simulink model "Microgrid_PV_WG_Bat_EV_j_22b"  (R2022b)
settings: Solver=VariableStepAuto  StartTime=0.0  StopTime=1  RelTol=1e-3
undefined symbols (not defined in the file or in its folder): Acid, Ion, Lead, Lithium
libraries: slpidlib x35, spsabctodq0Lib x23, spsSeriesRLCBranchLib x19, spsCurrentMeasurementLib x13, spsVoltageMeasurementLib x11, spsThreePhaseVIMeasurementLib x10, spsPLL3phLib x9, spsThreePhaseSeriesRLCBranchLib x9, spsPower3phInstantaneousLib x8, spsIGBTDiodeLib x8, spsUniversalBridgeLib x7, spsPWMGeneratorDCDCLib x6
(part 3 of 5)

== system Microgrid_PV_WG_Bat_EV_j_22b/Subsystem/电流内环控制，控制电网电流和电压同相 ==
  Id_ref : Inport
  Vd : Inport  Port=2
  Vq : Inport  Port=3
  f : Inport  Port=4
  Iq : Inport  Port=5
  Id : Inport  Port=6
  wt : Inport  Port=7
  Constant1 : Constant  Value=3e-3
  Constant2 : Constant  Value=0
  Constant3 : Constant  Value=0
  Constant4 : Constant  Value=3e-3
  Gain1 : Gain  Gain=2*pi
  Gain2 : Gain  Gain=2*pi
  Mux1 : Mux  Inputs=3
  PID Controller : slpidlib/PID Controller  Controller=PID  Form=Parallel  TimeDomain=Continuous-time  UseExternalTs=off  SampleTime=-1  IntegratorMethod=Forward Euler  FilterMethod=Forward Euler  ControllerParametersSource=internal  P=10  I=500  UseKiTs=off  D=0.5  N=100  UseFilter=on  TunerSelectOption=Transfer Function Based (PID Tuner App)  InitialConditionSource=internal  InitialConditionForIntegrator=0  InitialConditionForFilter=0  DifferentiatorICPrevScaledInput=0  ExternalReset=none  TrackingMode=off  Kt=1  LimitOutput=off  SatLimitsSource=internal  UpperSaturationLimit=inf  LowerSaturationLimit=-inf  LinearizeAsGain=on  AntiWindupMode=none  Kb=1  LimitIntegrator=off  UpperIntegratorSaturationLimit=inf  LowerIntegratorSaturationLimit=-inf  POutMin=[]  POutMax=[]  IOutMin=[]  IOutMax=[]  DOutMin=[]  DOutMax=[]  NOutMin=[]  NOutMax=[]  SumOutMin=[]  SumOutMax=[]  SaturationOutMin=[]  SaturationOutMax=[]  PParamMin=[]  PParamMax=[]  IParamMin=[]  IParamMax=[]  DParamMin=[]  DParamMax=[]  NParamMin=[]  NParamMax=[]  KbParamMin=[]  KbParamMax=[]  KtParamMin=[]  KtParamMax=[]  KbOutMin=[]  KbOutMax=[]  KtOutMin=[]  KtOutMax=[]  IntegratorOutMin=[]  IntegratorOutMax=[]  FilterOutMin=[]  FilterOutMax=[]  SumI1OutMin=[]  SumI1OutMax=[]  SumI2OutMin=[]  SumI2OutMax=[]  SumI3OutMin=[]  SumI3OutMax=[]  SumI4OutMin=[]  SumI4OutMax=[]  SumDOutMin=[]  SumDOutMax=[]  DifferentiatorOutMin=[]  DifferentiatorOutMax=[]  FilterDiffOutCoefMin=[]  FilterDiffOutCoefMax=[]  ReciprocalOutMin=[]  ReciprocalOutMax=[]  SumDenOutMin=[]  SumDenOutMax=[]  SumNumOutMin=[]  SumNumOutMax=[]  DivideOutMin=[]  DivideOutMax=[]  UdiffTsProdOutMin=[]  UdiffTsProdOutMax=[]  NTsProdOutMin=[]  NTsProdOutMax=[]  UintegralTsProdOutMin=[]  UintegralTsProdOutMax=[]  UngainTsProdOutMin=[]  UngainTsProdOutMax=[]  IntegratorContinuousStateAttributes=''  IntegratorStateMustResolveToSignalObject=off  IntegratorRTWStateStorageClass=Auto  FilterContinuousStateAttributes=''  FilterStateMustResolveToSignalObject=off  FilterRTWStateStorageClass=Auto  ParallelPVariant=InternalParameters  IdealPVariant=Disabled  IVariant=InternalParameters  DVariant=InternalParameters  IntegratorVariant=Continuous  SatVariant=Disabled  AWVariant=Passthrough  PCopyVariant=Disabled  TRVariant=Disabled  FdbkBlocksVariant=Forward  IdealPFdbkVariant=Disabled  SatFdbkVariant=Disabled  DerivativeFilterVariant=ContFilter  NVariant=InternalParameters  NCopyVariant=Disabled  FilterICVariant=InternalICsFilter  IntegratorICVariant=InternalICs  ExternalResetVariant=Disabled  TRSumVariant=Passthrough  SumFdbkVariant=Disabled  SumVariant=Sum_PID  TsampFilterVariant=InternalTs  TsampNgainVariant=Passthrough  TsampIntegralVariant=Disabled_SignalSpec  ExternalSaturationOutDataTypeStr=Inherit: Same as second input
  PID Controller1 : slpidlib/PID Controller  Controller=PID  Form=Parallel  TimeDomain=Continuous-time  UseExternalTs=off  SampleTime=-1  IntegratorMethod=Forward Euler  FilterMethod=Forward Euler  ControllerParametersSource=internal  P=10  I=500  UseKiTs=off  D=0.5  N=100  UseFilter=on  TunerSelectOption=Transfer Function Based (PID Tuner App)  InitialConditionSource=internal  InitialConditionForIntegrator=0  InitialConditionForFilter=0  DifferentiatorICPrevScaledInput=0  ExternalReset=none  TrackingMode=off  Kt=1  LimitOutput=off  SatLimitsSource=internal  UpperSaturationLimit=inf  LowerSaturationLimit=-inf  LinearizeAsGain=on  AntiWindupMode=none  Kb=1  LimitIntegrator=off  UpperIntegratorSaturationLimit=inf  LowerIntegratorSaturationLimit=-inf  POutMin=[]  POutMax=[]  IOutMin=[]  IOutMax=[]  DOutMin=[]  DOutMax=[]  NOutMin=[]  NOutMax=[]  SumOutMin=[]  SumOutMax=[]  SaturationOutMin=[]  SaturationOutMax=[]  PParamMin=[]  PParamMax=[]  IParamMin=[]  IParamMax=[]  DParamMin=[]  DParamMax=[]  NParamMin=[]  NParamMax=[]  KbParamMin=[]  KbParamMax=[]  KtParamMin=[]  KtParamMax=[]  KbOutMin=[]  KbOutMax=[]  KtOutMin=[]  KtOutMax=[]  IntegratorOutMin=[]  IntegratorOutMax=[]  FilterOutMin=[]  FilterOutMax=[]  SumI1OutMin=[]  SumI1OutMax=[]  SumI2OutMin=[]  SumI2OutMax=[]  SumI3OutMin=[]  SumI3OutMax=[]  SumI4OutMin=[]  SumI4OutMax=[]  SumDOutMin=[]  SumDOutMax=[]  DifferentiatorOutMin=[]  DifferentiatorOutMax=[]  FilterDiffOutCoefMin=[]  FilterDiffOutCoefMax=[]  ReciprocalOutMin=[]  ReciprocalOutMax=[]  SumDenOutMin=[]  SumDenOutMax=[]  SumNumOutMin=[]  SumNumOutMax=[]  DivideOutMin=[]  DivideOutMax=[]  UdiffTsProdOutMin=[]  UdiffTsProdOutMax=[]  NTsProdOutMin=[]  NTsProdOutMax=[]  UintegralTsProdOutMin=[]  UintegralTsProdOutMax=[]  UngainTsProdOutMin=[]  UngainTsProdOutMax=[]  IntegratorContinuousStateAttributes=''  IntegratorStateMustResolveToSignalObject=off  IntegratorRTWStateStorageClass=Auto  FilterContinuousStateAttributes=''  FilterStateMustResolveToSignalObject=off  FilterRTWStateStorageClass=Auto  ParallelPVariant=InternalParameters  IdealPVariant=Disabled  IVariant=InternalParameters  DVariant=InternalParameters  IntegratorVariant=Continuous  SatVariant=Disabled  AWVariant=Passthrough  PCopyVariant=Disabled  TRVariant=Disabled  FdbkBlocksVariant=Forward  IdealPFdbkVariant=Disabled  SatFdbkVariant=Disabled  DerivativeFilterVariant=ContFilter  NVariant=InternalParameters  NCopyVariant=Disabled  FilterICVariant=InternalICsFilter  IntegratorICVariant=InternalICs  ExternalResetVariant=Disabled  TRSumVariant=Passthrough  SumFdbkVariant=Disabled  SumVariant=Sum_PID  TsampFilterVariant=InternalTs  TsampNgainVariant=Passthrough  TsampIntegralVariant=Disabled_SignalSpec  ExternalSaturationOutDataTypeStr=Inherit: Same as second input
  PWM Generator (2-Level) : spsPWMGenerator2LevelLib/PWM Generator (2-Level)  ModulatorType=Three-phase bridge (6 pulses)  ModulatorMode=Unsynchronized  Fc=27*60  Pc=90  nF=27  MinMax="[ -1  1 ]"  SamplingTechnique=Natural  ModulatingSignals=off  m=0.8  Freq=60  Phase=0  Ts=0  ShowCarrierOutport=off
  Product{,1..3} (4 alike) : Product
  Subtract1 : Sum  Inputs=+-
  Subtract2 : Sum  Inputs=+-
  Sum : Sum  Inputs=+++
  Sum1 : Sum  Inputs=++-
  dq0 to abc : spsdq0toabcLib/dq0 to abc  Alignment=90 degrees behind phase A axis
  P : Outport
  wires:
  Gain2/1 -> Product2/1
  PWM Generator (2-Level)/1 -> P/1
  Constant4/1 -> Product2/2
  Mux1/1 -> dq0 to abc/1
  Sum/1 -> Mux1/1  "ud*"
  Id_ref/1 -> Subtract2/1
  Sum1/1 -> Mux1/2  "uq*"
  Product2/1 -> Product3/1
  dq0 to abc/1 -> PWM Generator (2-Level)/1
  Constant2/1 -> Subtract1/1  "iq*"
  Subtract2/1 -> PID Controller/1
  Constant3/1 -> Mux1/3
  PID Controller/1 -> Sum/2
  Vq/1 -> Sum1/1
  Product1/1 -> Sum/1
  Iq/1 -> Product1/2, Subtract1/2
  Constant1/1 -> Product/2
  f/1 -> Gain2/1, Gain1/1
  Gain1/1 -> Product/1
  wt/1 -> dq0 to abc/2
  Subtract1/1 -> PID Controller1/1
  Product3/1 -> Sum1/3
  PID Controller1/1 -> Sum1/2
  Product/1 -> Product1/1
  Id/1 -> Product3/2, Subtract2/2
  Vd/1 -> Sum/3

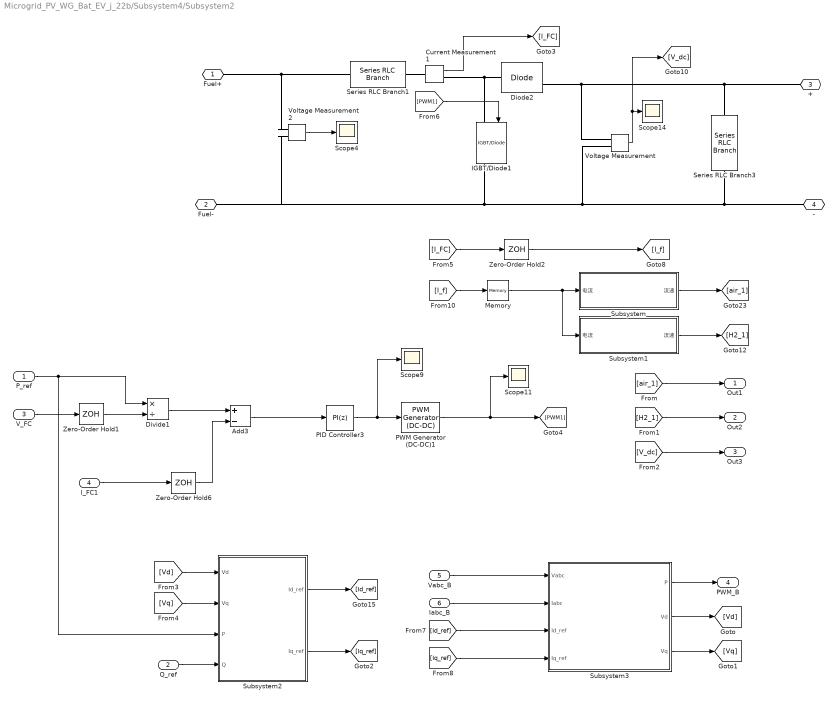
== system Microgrid_PV_WG_Bat_EV_j_22b/Subsystem4/Subsystem2 ==
  P_ref : Inport
  Q_ref : Inport  Port=2
  V_FC : Inport  Port=3
  I_FC1 : Inport  Port=4
  Vabc_B : Inport  Port=5
  Iabc_B : Inport  Port=6
  Add3 : Sum  Inputs=+-
  Current Measurement1 : spsCurrentMeasurementLib/Current Measurement  PhasorSimulation=off  OutputType=Complex  PSBequivalent=0
  Diode2 : spsDiodeLib/Diode  Ron=0.001  Lon=0  Vf=0.8  IC=0  UseSnubber=0  Rs=500  Cs=250e-9  Measurements=on
  Divide1 : Product  Inputs=*/
  IGBT/Diode1 : spsIGBTDiodeLib/IGBT//Diode  Ron=1e-3  Rs=1e5  Cs=inf  Measurements=on
  Memory : Memory  InitialCondition=1
  PID Controller3 : slpidlib/PID Controller  Controller=PI  Form=Parallel  TimeDomain=Discrete-time  UseExternalTs=off  SampleTime=-1  IntegratorMethod=Forward Euler  FilterMethod=Forward Euler  ControllerParametersSource=internal  P=1  I=1  UseKiTs=off  D=0  N=100  UseFilter=on  TunerSelectOption=Transfer Function Based (PID Tuner App)  InitialConditionSource=internal  InitialConditionForIntegrator=0  InitialConditionForFilter=0  DifferentiatorICPrevScaledInput=0  ExternalReset=none  TrackingMode=off  Kt=1  LimitOutput=off  SatLimitsSource=internal  UpperSaturationLimit=inf  LowerSaturationLimit=-inf  LinearizeAsGain=on  AntiWindupMode=none  Kb=1  LimitIntegrator=off  UpperIntegratorSaturationLimit=inf  LowerIntegratorSaturationLimit=-inf  POutMin=[]  POutMax=[]  IOutMin=[]  IOutMax=[]  DOutMin=[]  DOutMax=[]  NOutMin=[]  NOutMax=[]  SumOutMin=[]  SumOutMax=[]  SaturationOutMin=[]  SaturationOutMax=[]  PParamMin=[]  PParamMax=[]  IParamMin=[]  IParamMax=[]  DParamMin=[]  DParamMax=[]  NParamMin=[]  NParamMax=[]  KbParamMin=[]  KbParamMax=[]  KtParamMin=[]  KtParamMax=[]  KbOutMin=[]  KbOutMax=[]  KtOutMin=[]  KtOutMax=[]  IntegratorOutMin=[]  IntegratorOutMax=[]  FilterOutMin=[]  FilterOutMax=[]  SumI1OutMin=[]  SumI1OutMax=[]  SumI2OutMin=[]  SumI2OutMax=[]  SumI3OutMin=[]  SumI3OutMax=[]  SumI4OutMin=[]  SumI4OutMax=[]  SumDOutMin=[]  SumDOutMax=[]  DifferentiatorOutMin=[]  DifferentiatorOutMax=[]  FilterDiffOutCoefMin=[]  FilterDiffOutCoefMax=[]  ReciprocalOutMin=[]  ReciprocalOutMax=[]  SumDenOutMin=[]  SumDenOutMax=[]  SumNumOutMin=[]  SumNumOutMax=[]  DivideOutMin=[]  DivideOutMax=[]  UdiffTsProdOutMin=[]  UdiffTsProdOutMax=[]  NTsProdOutMin=[]  NTsProdOutMax=[]  UintegralTsProdOutMin=[]  UintegralTsProdOutMax=[]  UngainTsProdOutMin=[]  UngainTsProdOutMax=[]  IntegratorContinuousStateAttributes=''  IntegratorStateMustResolveToSignalObject=off  IntegratorRTWStateStorageClass=Auto  FilterContinuousStateAttributes=''  FilterStateMustResolveToSignalObject=off  FilterRTWStateStorageClass=Auto  ParallelPVariant=InternalParameters  IdealPVariant=Disabled  IVariant=InternalParameters  DVariant=Disabled  IntegratorVariant=Discrete  SatVariant=Disabled  AWVariant=Passthrough  PCopyVariant=Disabled  TRVariant=Disabled  FdbkBlocksVariant=Forward  IdealPFdbkVariant=Disabled  SatFdbkVariant=Disabled  DerivativeFilterVariant=Disabled  NVariant=Disabled  NCopyVariant=Disabled_SignalSpec  FilterICVariant=Disabled  IntegratorICVariant=InternalICs  ExternalResetVariant=Disabled  TRSumVariant=Passthrough  SumFdbkVariant=Disabled  SumVariant=Sum_PI  TsampFilterVariant=InternalTs  TsampNgainVariant=Passthrough  TsampIntegralVariant=Disabled_SignalSpec  ExternalSaturationOutDataTypeStr=Inherit: Same as second input
  PWM Generator (DC-DC)1 : spsPWMGeneratorDCDCLib/PWM Generator (DC-DC)  Fsw=1e4  Ts=0
  Scope{4,9,11,14} (4 alike) : Scope
  Series RLC Branch1 : spsSeriesRLCBranchLib/Series RLC Branch  LConnTagsString=__new0  RConnTagsString=__new0  BranchType=L  Resistance=1  Inductance=1e-2  SetiL0=off  InitialCurrent=0  Capacitance=1e-6  Setx0=off  InitialVoltage=0  Measurements=None
  Series RLC Branch3 : spsSeriesRLCBranchLib/Series RLC Branch  LConnTagsString=__new0  RConnTagsString=__new0  BranchType=C  Resistance=1  Inductance=1e-3  SetiL0=off  InitialCurrent=0  Capacitance=5e-2  Setx0=on  InitialVoltage=1000  Measurements=None
  Subsystem : Subsystem  mask{T=65, N=65, P=1.5, Uf_H2=99.56, x=99.95}
      mask prompts: T "温度"; N "数量"; P "氢气压强"; Uf_H2 "氢气利用率"; x "氢气百分比"
      mask DialogControl ParameterGroupVar Prompt: 参数
  Subsystem1 : Subsystem  mask{T=65, N=65, P=1, Uf_H2=59.3, x=21}
      mask prompts: T "温度"; N "数量"; P "氧气压强"; Uf_H2 "氧气利用率"; x "氧气百分比"
      mask DialogControl ParameterGroupVar Prompt: 参数
  Subsystem2 : Subsystem
  Subsystem3 : Subsystem
  Voltage Measurement : spsVoltageMeasurementLib/Voltage Measurement  PhasorSimulation=off  OutputType=Complex  PSBequivalent=0
  Voltage Measurement2 : spsVoltageMeasurementLib/Voltage Measurement  PhasorSimulation=off  OutputType=Complex  PSBequivalent=0
  Zero-Order Hold1 : ZeroOrderHold  SampleTime=1e-5
  Zero-Order Hold2 : ZeroOrderHold  SampleTime=1e-5
  Zero-Order Hold6 : ZeroOrderHold  SampleTime=1e-5
  Fuel+ : PMIOPort  Side=Left
  Fuel- : PMIOPort  Port=2  Side=Left
  + : PMIOPort  Port=3  Side=Right
  - : PMIOPort  Port=4  Side=Right
  Out1 : Outport
  Out2 : Outport  Port=2
  Out3 : Outport  Port=3
  PWM_B : Outport  Port=4
  wires:
  [PWM1] -> IGBT/Diode1/1
  Current Measurement1/1 -> [I_FC]
  Voltage Measurement/1 -> [V_dc], Scope14/1
  Voltage Measurement2/1 -> Scope4/1
  [I_FC] -> Zero-Order Hold2/1
  Zero-Order Hold2/1 -> [I_f]
  Subsystem/1(流速) -> [air_1]
  Subsystem1/1(流速) -> [H2_1]
  Memory/1 -> Subsystem1/1(电流), Subsystem/1(电流)
  [I_f] -> Memory/1
  [air_1] -> Out1/1
  [H2_1] -> Out2/1
  [V_dc] -> Out3/1
  Zero-Order Hold6/1 -> Add3/2
  Zero-Order Hold1/1 -> Divide1/2
  Divide1/1 -> Add3/1
  PWM Generator (DC-DC)1/1 -> Scope11/1, [PWM1]
  P_ref/1 -> Subsystem2/3(P), Divide1/1
  I_FC1/1 -> Zero-Order Hold6/1
  V_FC/1 -> Zero-Order Hold1/1
  Add3/1 -> PID Controller3/1
  PID Controller3/1 -> Scope9/1, PWM Generator (DC-DC)1/1
  Vabc_B/1 -> Subsystem3/1(Vabc)
  Iabc_B/1 -> Subsystem3/2(Iabc)
  Subsystem3/1(P) -> PWM_B/1
  Subsystem3/2(Vd) -> [Vd]
  Subsystem3/3(Vq) -> [Vq]
  [Vd] -> Subsystem2/1(Vd)
  [Vq] -> Subsystem2/2(Vq)
  Q_ref/1 -> Subsystem2/4(Q)
  Subsystem2/1(Id_ref) -> [Id_ref]
  Subsystem2/2(Iq_ref) -> [Iq_ref]
  [Id_ref] -> Subsystem3/3(Id_ref)
  [Iq_ref] -> Subsystem3/4(Iq_ref)
  connections:
  Current Measurement1/RConn1 -- IGBT/Diode1/LConn1 -- Diode2/LConn1
  Voltage Measurement2/LConn1 -- Fuel+/RConn1 -- Series RLC Branch1/LConn1
  Series RLC Branch3/LConn1 -- Voltage Measurement/LConn1 -- Diode2/RConn1 -- +/RConn1
  Current Measurement1/LConn1 -- Series RLC Branch1/RConn1
  IGBT/Diode1/RConn1 -- Voltage Measurement/LConn2 -- Series RLC Branch3/RConn1 -- -/RConn1 -- Voltage Measurement2/LConn2 -- Fuel-/RConn1

== system Microgrid_PV_WG_Bat_EV_j_22b/Subsystem4/Subsystem3 ==
  V_dc : Inport
  V_ref : Inport  Port=2
  Add1 : Sum  Inputs=+-
  Add4 : Sum  Inputs=+-
  Battery : spsBatteryLib/Battery  BatType=Lithium-Ion  ShowTempParam=off  ThermalPreset=no  ShowAgeParam=off  NomV=500  NomQ=100  SOC=50  Batt_Tr=30  PresetModel=on  MaxQ=100  MinV=375  FullV=581.9936  Dis_rate=43.4783  R=0.05  Normal_OP=90.4348  expZone="[540.1929      4.913043]"  current=[10 100]  Units=Time  Tci=20  NomT=20  T2=-30  MaxQ2=4.8  FullV2=7.1  Normal_OP2=5.655  expZone2="[6.58           1]"  Rca=0.6  ti=2000  Dp=0  Neq0=0  Tsim=1e6  Ta1=25  Qeol=5.4*0.9  Reol=0.013333*1.2  Char_age=[2.3478, 3]  Dis_age=[2.3478, 10]  N1=1500  N2=10500  N3=1000  N4=1400  Ta2=45  N5=950
  Current Measurement2 : spsCurrentMeasurementLib/Current Measurement  PhasorSimulation=off  OutputType=Complex  PSBequivalent=0
  Demux : Demux  Outputs=3
  IGBT/Diode2 : spsIGBTDiodeLib/IGBT//Diode  Ron=1e-3  Rs=1e5  Cs=inf  Measurements=on
  IGBT/Diode3 : spsIGBTDiodeLib/IGBT//Diode  Ron=1e-3  Rs=1e5  Cs=inf  Measurements=on
  NOT : Logic  Operator=NOT  IconShape=distinctive  AllPortsSameDT=off  OutDataTypeStr=boolean
  PID Controller2 : slpidlib/PID Controller  Controller=PI  Form=Parallel  TimeDomain=Continuous-time  UseExternalTs=off  SampleTime=-1  IntegratorMethod=Forward Euler  FilterMethod=Forward Euler  ControllerParametersSource=internal  P=10  I=1000  UseKiTs=off  D=0  N=100  UseFilter=on  TunerSelectOption=Transfer Function Based (PID Tuner App)  InitialConditionSource=internal  InitialConditionForIntegrator=0  InitialConditionForFilter=0  DifferentiatorICPrevScaledInput=0  ExternalReset=none  TrackingMode=off  Kt=1  LimitOutput=off  SatLimitsSource=internal  UpperSaturationLimit=inf  LowerSaturationLimit=-inf  LinearizeAsGain=on  AntiWindupMode=none  Kb=1  LimitIntegrator=off  UpperIntegratorSaturationLimit=inf  LowerIntegratorSaturationLimit=-inf  POutMin=[]  POutMax=[]  IOutMin=[]  IOutMax=[]  DOutMin=[]  DOutMax=[]  NOutMin=[]  NOutMax=[]  SumOutMin=[]  SumOutMax=[]  SaturationOutMin=[]  SaturationOutMax=[]  PParamMin=[]  PParamMax=[]  IParamMin=[]  IParamMax=[]  DParamMin=[]  DParamMax=[]  NParamMin=[]  NParamMax=[]  KbParamMin=[]  KbParamMax=[]  KtParamMin=[]  KtParamMax=[]  KbOutMin=[]  KbOutMax=[]  KtOutMin=[]  KtOutMax=[]  IntegratorOutMin=[]  IntegratorOutMax=[]  FilterOutMin=[]  FilterOutMax=[]  SumI1OutMin=[]  SumI1OutMax=[]  SumI2OutMin=[]  SumI2OutMax=[]  SumI3OutMin=[]  SumI3OutMax=[]  SumI4OutMin=[]  SumI4OutMax=[]  SumDOutMin=[]  SumDOutMax=[]  DifferentiatorOutMin=[]  DifferentiatorOutMax=[]  FilterDiffOutCoefMin=[]  FilterDiffOutCoefMax=[]  ReciprocalOutMin=[]  ReciprocalOutMax=[]  SumDenOutMin=[]  SumDenOutMax=[]  SumNumOutMin=[]  SumNumOutMax=[]  DivideOutMin=[]  DivideOutMax=[]  UdiffTsProdOutMin=[]  UdiffTsProdOutMax=[]  NTsProdOutMin=[]  NTsProdOutMax=[]  UintegralTsProdOutMin=[]  UintegralTsProdOutMax=[]  UngainTsProdOutMin=[]  UngainTsProdOutMax=[]  IntegratorContinuousStateAttributes=''  IntegratorStateMustResolveToSignalObject=off  IntegratorRTWStateStorageClass=Auto  FilterContinuousStateAttributes=''  FilterStateMustResolveToSignalObject=off  FilterRTWStateStorageClass=Auto  ParallelPVariant=InternalParameters  IdealPVariant=Disabled  IVariant=InternalParameters  DVariant=Disabled  IntegratorVariant=Continuous  SatVariant=Disabled  AWVariant=Passthrough  PCopyVariant=Disabled  TRVariant=Disabled  FdbkBlocksVariant=Forward  IdealPFdbkVariant=Disabled  SatFdbkVariant=Disabled  DerivativeFilterVariant=Disabled  NVariant=Disabled  NCopyVariant=Disabled_SignalSpec  FilterICVariant=Disabled  IntegratorICVariant=InternalICs  ExternalResetVariant=Disabled  TRSumVariant=Passthrough  SumFdbkVariant=Disabled  SumVariant=Sum_PI  TsampFilterVariant=InternalTs  TsampNgainVariant=Passthrough  TsampIntegralVariant=Disabled_SignalSpec  ExternalSaturationOutDataTypeStr=Inherit: Same as second input
  PID Controller4 : slpidlib/PID Controller  Controller=PI  Form=Parallel  TimeDomain=Continuous-time  UseExternalTs=off  SampleTime=-1  IntegratorMethod=Forward Euler  FilterMethod=Forward Euler  ControllerParametersSource=internal  P=1  I=1  UseKiTs=off  D=0  N=100  UseFilter=on  TunerSelectOption=Transfer Function Based (PID Tuner App)  InitialConditionSource=internal  InitialConditionForIntegrator=0  InitialConditionForFilter=0  DifferentiatorICPrevScaledInput=0  ExternalReset=none  TrackingMode=off  Kt=1  LimitOutput=off  SatLimitsSource=internal  UpperSaturationLimit=inf  LowerSaturationLimit=-inf  LinearizeAsGain=on  AntiWindupMode=none  Kb=1  LimitIntegrator=off  UpperIntegratorSaturationLimit=inf  LowerIntegratorSaturationLimit=-inf  POutMin=[]  POutMax=[]  IOutMin=[]  IOutMax=[]  DOutMin=[]  DOutMax=[]  NOutMin=[]  NOutMax=[]  SumOutMin=[]  SumOutMax=[]  SaturationOutMin=[]  SaturationOutMax=[]  PParamMin=[]  PParamMax=[]  IParamMin=[]  IParamMax=[]  DParamMin=[]  DParamMax=[]  NParamMin=[]  NParamMax=[]  KbParamMin=[]  KbParamMax=[]  KtParamMin=[]  KtParamMax=[]  KbOutMin=[]  KbOutMax=[]  KtOutMin=[]  KtOutMax=[]  IntegratorOutMin=[]  IntegratorOutMax=[]  FilterOutMin=[]  FilterOutMax=[]  SumI1OutMin=[]  SumI1OutMax=[]  SumI2OutMin=[]  SumI2OutMax=[]  SumI3OutMin=[]  SumI3OutMax=[]  SumI4OutMin=[]  SumI4OutMax=[]  SumDOutMin=[]  SumDOutMax=[]  DifferentiatorOutMin=[]  DifferentiatorOutMax=[]  FilterDiffOutCoefMin=[]  FilterDiffOutCoefMax=[]  ReciprocalOutMin=[]  ReciprocalOutMax=[]  SumDenOutMin=[]  SumDenOutMax=[]  SumNumOutMin=[]  SumNumOutMax=[]  DivideOutMin=[]  DivideOutMax=[]  UdiffTsProdOutMin=[]  UdiffTsProdOutMax=[]  NTsProdOutMin=[]  NTsProdOutMax=[]  UintegralTsProdOutMin=[]  UintegralTsProdOutMax=[]  UngainTsProdOutMin=[]  UngainTsProdOutMax=[]  IntegratorContinuousStateAttributes=''  IntegratorStateMustResolveToSignalObject=off  IntegratorRTWStateStorageClass=Auto  FilterContinuousStateAttributes=''  FilterStateMustResolveToSignalObject=off  FilterRTWStateStorageClass=Auto  ParallelPVariant=InternalParameters  IdealPVariant=Disabled  IVariant=InternalParameters  DVariant=Disabled  IntegratorVariant=Continuous  SatVariant=Disabled  AWVariant=Passthrough  PCopyVariant=Disabled  TRVariant=Disabled  FdbkBlocksVariant=Forward  IdealPFdbkVariant=Disabled  SatFdbkVariant=Disabled  DerivativeFilterVariant=Disabled  NVariant=Disabled  NCopyVariant=Disabled_SignalSpec  FilterICVariant=Disabled  IntegratorICVariant=InternalICs  ExternalResetVariant=Disabled  TRSumVariant=Passthrough  SumFdbkVariant=Disabled  SumVariant=Sum_PI  TsampFilterVariant=InternalTs  TsampNgainVariant=Passthrough  TsampIntegralVariant=Disabled_SignalSpec  ExternalSaturationOutDataTypeStr=Inherit: Same as second input
  PWM Generator (DC-DC)2 : spsPWMGeneratorDCDCLib/PWM Generator (DC-DC)  Fsw=1e4  Ts=0
  Scope : Scope  NumInputPorts=3
  Series RLC Branch4 : spsSeriesRLCBranchLib/Series RLC Branch  LConnTagsString=__new0  RConnTagsString=__new0  BranchType=L  Resistance=1  Inductance=1e-3  SetiL0=off  InitialCurrent=0  Capacitance=1e-6  Setx0=off  InitialVoltage=0  Measurements=None
  Series RLC Branch5 : spsSeriesRLCBranchLib/Series RLC Branch  LConnTagsString=__new0  RConnTagsString=__new0  BranchType=C  Resistance=1  Inductance=1e-3  SetiL0=off  InitialCurrent=0  Capacitance=1e-3  Setx0=off  InitialVoltage=0  Measurements=None
  Series RLC Branch6 : spsSeriesRLCBranchLib/Series RLC Branch  LConnTagsString=__new0  RConnTagsString=__new0  BranchType=R  Resistance=1  Inductance=1e-3  SetiL0=off  InitialCurrent=0  Capacitance=1e-6  Setx0=off  InitialVoltage=0  Measurements=None
  Zero-Order Hold4 : ZeroOrderHold  SampleTime=1e-5
  Zero-Order Hold5 : ZeroOrderHold  SampleTime=1e-5
  Bat+ : PMIOPort  Side=Left
  Bat- : PMIOPort  Port=2  Side=Left
  Out1 : Outport
  wires:
  Current Measurement2/1 -> [I_BA]
  [PWM2] -> IGBT/Diode2/1
  [PWM3] -> IGBT/Diode3/1
  PID Controller2/1 -> Add4/1
  Add1/1 -> PID Controller2/1
  Zero-Order Hold5/1 -> Add1/1
  PWM Generator (DC-DC)2/1 -> NOT/1, [PWM2]
  PID Controller4/1 -> PWM Generator (DC-DC)2/1
  Add4/1 -> PID Controller4/1
  NOT/1 -> [PWM3]
  V_ref/1 -> Add1/2
  [I_BA] -> Zero-Order Hold4/1
  Zero-Order Hold4/1 -> Add4/2
  V_dc/1 -> Zero-Order Hold5/1
  Battery/1 -> Demux/1
  Demux/1 -> Scope/1
  Demux/2 -> Scope/2
  Demux/3 -> Scope/3
  connections:
  Current Measurement2/RConn1 -- Battery/LConn1 -- Series RLC Branch6/LConn1
  IGBT/Diode3/RConn1 -- Series RLC Branch5/RConn1 -- Battery/LConn2 -- Series RLC Branch6/RConn1 -- Bat-/RConn1
  IGBT/Diode3/LConn1 -- IGBT/Diode2/RConn1 -- Series RLC Branch4/LConn1
  Series RLC Branch5/LConn1 -- Current Measurement2/LConn1 -- Series RLC Branch4/RConn1
  IGBT/Diode2/LConn1 -- Bat+/RConn1

== system Microgrid_PV_WG_Bat_EV_j_22b/储氢罐/氢气消耗速率转换 ==
  L/min : Inport
  Add : Sum
  Divide : Product  Inputs=*/
  Gain : Gain  Gain=1/60/1000
  P : Constant  Value=101325
  Product : Product
  Product1 : Product
  R : Constant  Value=8.314
  T/C : Constant  Value=25
  conversion : Constant  Value=273.15
  mol/s : Outport
  wires:
  P/1 -> Product/2
  conversion/1 -> Add/2
  T/C/1 -> Add/1
  R/1 -> Product1/1
  Add/1 -> Product1/2  "T/K"
  Product/1 -> Divide/1
  L/min/1 -> Gain/1
  Product1/1 -> Divide/2
  Gain/1 -> Product/1
  Divide/1 -> mol/s/1

== system Microgrid_PV_WG_Bat_EV_j_22b/充电桩/恒流恒压充电 ==
  V : Inport
  I : Inport  Port=2
  Add : Sum
  Constant : Constant
  Constant1 : Constant  Value=0
  Constant2 : Constant
  Memory : Memory
  Memory1 : Memory  InitialCondition=0.3
  Saturation : Saturate  UpperLimit=1  LowerLimit=0
  Sign : Signum
  Sum1 : Sum  Inputs=|++
  Sum2 : Sum  Inputs=|-+
  Switch : Switch  Threshold=500  SaturateOnIntegerOverflow=off  InputSameDT=off
  恒压 : Subsystem
  恒流 : Subsystem
  D : Outport
  wires:
  V/1 -> Switch/2, 恒压/1(V)
  恒压/1(I_out) -> Add/2
  I/1 -> 恒流/1(I)
  Add/1 -> Saturation/1
  Saturation/1 -> Memory1/1
  Constant/1 -> Switch/1
  Constant1/1 -> Switch/3
  Sum1/1 -> Memory/1
  Memory/1 -> Sign/1
  Sign/1 -> Sum2/1, 恒压/Enable, Sum1/2
  Switch/1 -> Sum1/1
  Constant2/1 -> Sum2/2
  Sum2/1 -> 恒流/Enable
  恒流/1(I_out) -> Add/1
  Memory1/1 -> D/1

== system Microgrid_PV_WG_Bat_EV_j_22b/光伏/电导增量法MPPT ==
  V : Inport
  I : Inport  Port=2
  Add : Sum
  Add1 : Sum
  Constant : Constant  Value=0
  Constant1 : Constant  Value=0
  Gain : Gain  Gain=-2e-6
  Gain1 : Gain  Gain=-2e-6
  Math Function : Math  Operator=square
  Memory : Memory
  Memory1 : Memory
  Memory2 : Memory  InitialCondition=0.5
  Product : Product  Inputs=3
  Product1 : Product
  Sign : Signum
  Sign1 : Signum
  Subtract : Sum  Inputs=+-
  Switch : Switch  Criteria=u2 ~= 0  SaturateOnIntegerOverflow=off  InputSameDT=off
  Switch1 : Switch  Criteria=u2 ~= 0  SaturateOnIntegerOverflow=off  InputSameDT=off
  Switch2 : Switch  Criteria=u2 ~= 0  SaturateOnIntegerOverflow=off  InputSameDT=off
  计算电流变化量 : Sum  Inputs=+-
  D : Outport
  wires:
  V/1 -> Product/3, Memory1/1, Subtract/1
  Memory/1 -> 计算电流变化量/2
  Memory1/1 -> Subtract/2
  Switch/1 -> Add/1
  Add/1 -> D/1, Memory2/1  "过程量转为状态量"
  Memory2/1 -> Add/2
  I/1 -> Product1/2, Memory/1, 计算电流变化量/1
  Subtract/1 -> Switch/2, Product/1, Math Function/1  "dV"
  Math Function/1 -> Product1/1
  计算电流变化量/1 -> Sign1/1, Product/2, Switch2/2  "dI"
  Product1/1 -> Add1/1
  Product/1 -> Add1/2
  Add1/1 -> Sign/1, Switch1/2  "I+dI/dV*V"
  Constant/1 -> Switch1/3
  Sign/1 -> Gain/1
  Gain/1 -> Switch1/1
  Switch1/1 -> Switch/1
  Constant1/1 -> Switch2/3
  Sign1/1 -> Gain1/1
  Gain1/1 -> Switch2/1
  Switch2/1 -> Switch/3

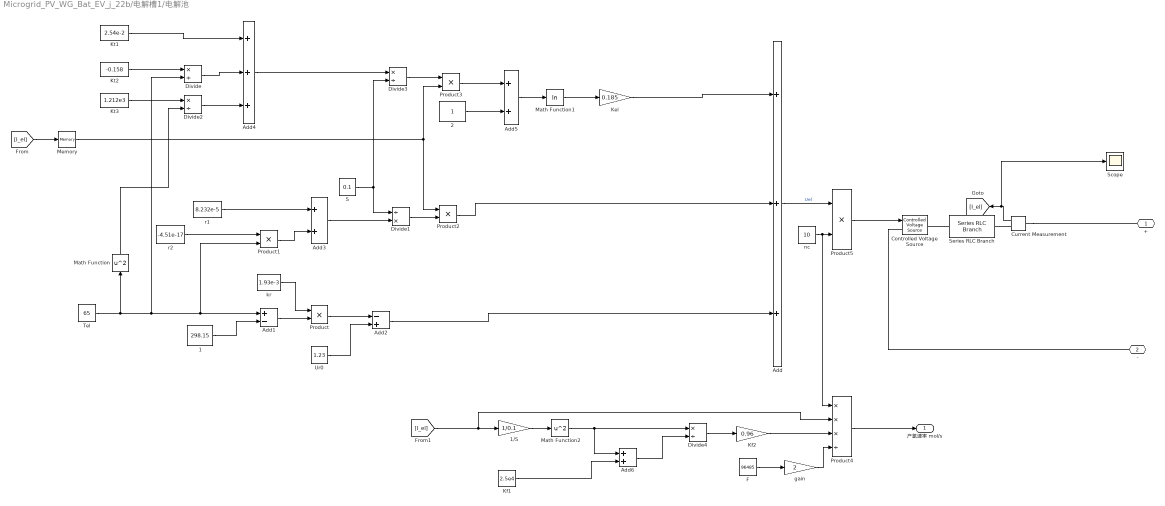
== system Microgrid_PV_WG_Bat_EV_j_22b/电解槽1/电解池 ==
  1 : Constant  Value=298.15
  1/S : Gain  Gain=1/0.1
  2 : Constant
  Add : Sum  Inputs=+++
  Add1 : Sum  Inputs=+-
  Add2 : Sum  Inputs=-+
  Add3 : Sum
  Add4 : Sum  Inputs=+++
  Add5 : Sum
  Add6 : Sum
  Controlled Voltage Source : spsControlledVoltageSourceLib/Controlled Voltage Source  Initialize=on  Source_Type=AC  Amplitude=0  Phase=0  Frequency=0  Measurements=None
  Current Measurement : spsCurrentMeasurementLib/Current Measurement  PhasorSimulation=off  OutputType=Complex  PSBequivalent=0
  Divide{,2..4} (4 alike) : Product  Inputs=*/
  Divide1 : Product  Inputs=/*
  F : Constant  Value=96485
  Kel : Gain  Gain=0.185
  Kf1 : Constant  Value=2.5e4
  Kf2 : Gain  Gain=0.96
  Kt1 : Constant  Value=2.54e-2
  Kt2 : Constant  Value=-0.158
  Kt3 : Constant  Value=1.212e3
  Math Function : Math  Operator=square
  Math Function1 : Math  Operator=log
  Math Function2 : Math  Operator=square
  Memory : Memory  InitialCondition=10
  Product{,1..3,5} (5 alike) : Product
  Product4 : Product  Inputs=***/
  S : Constant  Value=0.1
  Scope : Scope
  Series RLC Branch : spsSeriesRLCBranchLib/Series RLC Branch  LConnTagsString=__new0  RConnTagsString=__new0  BranchType=R  Resistance=1  Inductance=1e-3  SetiL0=off  InitialCurrent=0  Capacitance=1e-6  Setx0=off  InitialVoltage=0  Measurements=None
  Tel : Constant  Value=65
  Ur0 : Constant  Value=1.23
  gain : Gain  Gain=2
  kr : Constant  Value=1.93e-3
  nc : Constant  Value=10
  r1 : Constant  Value=8.232e-5
  r2 : Constant  Value=-4.51e-17
  + : PMIOPort  Side=Left
  - : PMIOPort  Port=2  Side=Left
  产氢速率 mol/s : Outport
  wires:
  Add3/1 -> Divide1/2
  Kt2/1 -> Divide/1
  Divide3/1 -> Product3/1
  Tel/1 -> Math Function/1, Divide/2, Product1/2, Add1/1
  [I_el] -> Memory/1
  Add5/1 -> Math Function1/1
  S/1 -> Divide3/2, Divide1/1
  Current Measurement/1 -> Scope/1, [I_el]
  r2/1 -> Product1/1
  Product1/1 -> Add3/2
  Product/1 -> Add2/1
  Math Function1/1 -> Kel/1
  1/1 -> Add1/2
  2/1 -> Add5/2
  r1/1 -> Add3/1
  Divide/1 -> Add4/2
  Add2/1 -> Add/3
  Kel/1 -> Add/1
  Add4/1 -> Divide3/1
  Product2/1 -> Add/2
  Kt3/1 -> Divide2/1
  Math Function/1 -> Divide2/2
  Kt1/1 -> Add4/1
  Divide2/1 -> Add4/3
  Ur0/1 -> Add2/2
  Divide1/1 -> Product2/2
  Product3/1 -> Add5/1
  Add1/1 -> Product/2
  kr/1 -> Product/1
  Add/1 -> Product5/1  "Uel"
  1/S/1 -> Math Function2/1
  Kf1/1 -> Add6/2
  Math Function2/1 -> Divide4/1, Add6/1
  Add6/1 -> Divide4/2
  [I_el] -> Product4/2, 1/S/1
  Divide4/1 -> Kf2/1
  Kf2/1 -> Product4/3
  nc/1 -> Product4/1, Product5/2
  Product5/1 -> Controlled Voltage Source/1
  F/1 -> gain/1
  gain/1 -> Product4/4
  Product4/1 -> 产氢速率 mol/s/1
  Memory/1 -> Product3/2, Product2/1
  connections:
  Controlled Voltage Source/LConn1 -- -/RConn1
  Series RLC Branch/LConn1 -- Controlled Voltage Source/RConn1
  Current Measurement/RConn1 -- Series RLC Branch/RConn1
  Current Measurement/LConn1 -- +/RConn1

== system Microgrid_PV_WG_Bat_EV_j_22b/逆变器整流/controller2 ==
  note: abc2dq
  Udc : Inport
  Udc_ref : Inport  Port=2
  Vabc : Inport  Port=3
  Iabc : Inport  Port=4
  Constant : Constant  Commented=on  Value=600
  Constant4 : Constant  Value=0
  Demux2 : Demux  Outputs=3
  Demux3 : Demux  Outputs=3
  Demux4 : Demux  Outputs=3
  Gain6 : Gain  Gain=2*pi*50*(7e-3)
  Gain7 : Gain  Gain=2*pi*50*(7e-3)
  Gain9 : Gain  Gain=0.0017
  Mux1 : Mux  Inputs=3
  PID 3 : slpidlib/PID Controller  Controller=PID  Form=Parallel  TimeDomain=Discrete-time  UseExternalTs=off  SampleTime=1e-5  IntegratorMethod=Forward Euler  FilterMethod=Forward Euler  ControllerParametersSource=internal  P=2  I=70  UseKiTs=off  D=0  N=100  UseFilter=on  TunerSelectOption=Transfer Function Based (PID Tuner App)  InitialConditionSource=internal  InitialConditionForIntegrator=0  InitialConditionForFilter=0  DifferentiatorICPrevScaledInput=0  ExternalReset=none  TrackingMode=off  Kt=1  LimitOutput=off  SatLimitsSource=internal  UpperSaturationLimit=inf  LowerSaturationLimit=-inf  LinearizeAsGain=on  AntiWindupMode=none  Kb=1  LimitIntegrator=off  UpperIntegratorSaturationLimit=inf  LowerIntegratorSaturationLimit=-inf  POutMin=[]  POutMax=[]  IOutMin=[]  IOutMax=[]  DOutMin=[]  DOutMax=[]  NOutMin=[]  NOutMax=[]  SumOutMin=[]  SumOutMax=[]  SaturationOutMin=[]  SaturationOutMax=[]  PParamMin=[]  PParamMax=[]  IParamMin=[]  IParamMax=[]  DParamMin=[]  DParamMax=[]  NParamMin=[]  NParamMax=[]  KbParamMin=[]  KbParamMax=[]  KtParamMin=[]  KtParamMax=[]  KbOutMin=[]  KbOutMax=[]  KtOutMin=[]  KtOutMax=[]  IntegratorOutMin=[]  IntegratorOutMax=[]  FilterOutMin=[]  FilterOutMax=[]  SumI1OutMin=[]  SumI1OutMax=[]  SumI2OutMin=[]  SumI2OutMax=[]  SumI3OutMin=[]  SumI3OutMax=[]  SumI4OutMin=[]  SumI4OutMax=[]  SumDOutMin=[]  SumDOutMax=[]  DifferentiatorOutMin=[]  DifferentiatorOutMax=[]  FilterDiffOutCoefMin=[]  FilterDiffOutCoefMax=[]  ReciprocalOutMin=[]  ReciprocalOutMax=[]  SumDenOutMin=[]  SumDenOutMax=[]  SumNumOutMin=[]  SumNumOutMax=[]  DivideOutMin=[]  DivideOutMax=[]  UdiffTsProdOutMin=[]  UdiffTsProdOutMax=[]  NTsProdOutMin=[]  NTsProdOutMax=[]  UintegralTsProdOutMin=[]  UintegralTsProdOutMax=[]  UngainTsProdOutMin=[]  UngainTsProdOutMax=[]  IntegratorContinuousStateAttributes=''  IntegratorStateMustResolveToSignalObject=off  IntegratorRTWStateStorageClass=Auto  FilterContinuousStateAttributes=''  FilterStateMustResolveToSignalObject=off  FilterRTWStateStorageClass=Auto  ParallelPVariant=InternalParameters  IdealPVariant=Disabled  IVariant=InternalParameters  DVariant=InternalParameters  IntegratorVariant=Discrete  SatVariant=Disabled  AWVariant=Passthrough  PCopyVariant=Disabled  TRVariant=Disabled  FdbkBlocksVariant=Forward  IdealPFdbkVariant=Disabled  SatFdbkVariant=Disabled  DerivativeFilterVariant=ForwardEulerFilter  NVariant=InternalParameters  NCopyVariant=Disabled  FilterICVariant=InternalICsFilter  IntegratorICVariant=InternalICs  ExternalResetVariant=Disabled  TRSumVariant=Passthrough  SumFdbkVariant=Disabled  SumVariant=Sum_PID  TsampFilterVariant=InternalTs  TsampNgainVariant=Passthrough  TsampIntegralVariant=Disabled_SignalSpec  ExternalSaturationOutDataTypeStr=Inherit: Same as second input
  PID 4 : slpidlib/PID Controller  Controller=PID  Form=Parallel  TimeDomain=Discrete-time  UseExternalTs=off  SampleTime=1e-5  IntegratorMethod=Forward Euler  FilterMethod=Forward Euler  ControllerParametersSource=internal  P=10  I=0  UseKiTs=off  D=0  N=100  UseFilter=on  TunerSelectOption=Transfer Function Based (PID Tuner App)  InitialConditionSource=internal  InitialConditionForIntegrator=0  InitialConditionForFilter=0  DifferentiatorICPrevScaledInput=0  ExternalReset=none  TrackingMode=off  Kt=1  LimitOutput=off  SatLimitsSource=internal  UpperSaturationLimit=inf  LowerSaturationLimit=-inf  LinearizeAsGain=on  AntiWindupMode=none  Kb=1  LimitIntegrator=off  UpperIntegratorSaturationLimit=inf  LowerIntegratorSaturationLimit=-inf  POutMin=[]  POutMax=[]  IOutMin=[]  IOutMax=[]  DOutMin=[]  DOutMax=[]  NOutMin=[]  NOutMax=[]  SumOutMin=[]  SumOutMax=[]  SaturationOutMin=[]  SaturationOutMax=[]  PParamMin=[]  PParamMax=[]  IParamMin=[]  IParamMax=[]  DParamMin=[]  DParamMax=[]  NParamMin=[]  NParamMax=[]  KbParamMin=[]  KbParamMax=[]  KtParamMin=[]  KtParamMax=[]  KbOutMin=[]  KbOutMax=[]  KtOutMin=[]  KtOutMax=[]  IntegratorOutMin=[]  IntegratorOutMax=[]  FilterOutMin=[]  FilterOutMax=[]  SumI1OutMin=[]  SumI1OutMax=[]  SumI2OutMin=[]  SumI2OutMax=[]  SumI3OutMin=[]  SumI3OutMax=[]  SumI4OutMin=[]  SumI4OutMax=[]  SumDOutMin=[]  SumDOutMax=[]  DifferentiatorOutMin=[]  DifferentiatorOutMax=[]  FilterDiffOutCoefMin=[]  FilterDiffOutCoefMax=[]  ReciprocalOutMin=[]  ReciprocalOutMax=[]  SumDenOutMin=[]  SumDenOutMax=[]  SumNumOutMin=[]  SumNumOutMax=[]  DivideOutMin=[]  DivideOutMax=[]  UdiffTsProdOutMin=[]  UdiffTsProdOutMax=[]  NTsProdOutMin=[]  NTsProdOutMax=[]  UintegralTsProdOutMin=[]  UintegralTsProdOutMax=[]  UngainTsProdOutMin=[]  UngainTsProdOutMax=[]  IntegratorContinuousStateAttributes=''  IntegratorStateMustResolveToSignalObject=off  IntegratorRTWStateStorageClass=Auto  FilterContinuousStateAttributes=''  FilterStateMustResolveToSignalObject=off  FilterRTWStateStorageClass=Auto  ParallelPVariant=InternalParameters  IdealPVariant=Disabled  IVariant=InternalParameters  DVariant=InternalParameters  IntegratorVariant=Discrete  SatVariant=Disabled  AWVariant=Passthrough  PCopyVariant=Disabled  TRVariant=Disabled  FdbkBlocksVariant=Forward  IdealPFdbkVariant=Disabled  SatFdbkVariant=Disabled  DerivativeFilterVariant=ForwardEulerFilter  NVariant=InternalParameters  NCopyVariant=Disabled  FilterICVariant=InternalICsFilter  IntegratorICVariant=InternalICs  ExternalResetVariant=Disabled  TRSumVariant=Passthrough  SumFdbkVariant=Disabled  SumVariant=Sum_PID  TsampFilterVariant=InternalTs  TsampNgainVariant=Passthrough  TsampIntegralVariant=Disabled_SignalSpec  ExternalSaturationOutDataTypeStr=Inherit: Same as second input
  PID 5 : slpidlib/PID Controller  Controller=PID  Form=Parallel  TimeDomain=Discrete-time  UseExternalTs=off  SampleTime=1e-5  IntegratorMethod=Forward Euler  FilterMethod=Forward Euler  ControllerParametersSource=internal  P=10  I=0  UseKiTs=off  D=0  N=100  UseFilter=on  TunerSelectOption=Transfer Function Based (PID Tuner App)  InitialConditionSource=internal  InitialConditionForIntegrator=0  InitialConditionForFilter=0  DifferentiatorICPrevScaledInput=0  ExternalReset=none  TrackingMode=off  Kt=1  LimitOutput=off  SatLimitsSource=internal  UpperSaturationLimit=inf  LowerSaturationLimit=-inf  LinearizeAsGain=on  AntiWindupMode=none  Kb=1  LimitIntegrator=off  UpperIntegratorSaturationLimit=inf  LowerIntegratorSaturationLimit=-inf  POutMin=[]  POutMax=[]  IOutMin=[]  IOutMax=[]  DOutMin=[]  DOutMax=[]  NOutMin=[]  NOutMax=[]  SumOutMin=[]  SumOutMax=[]  SaturationOutMin=[]  SaturationOutMax=[]  PParamMin=[]  PParamMax=[]  IParamMin=[]  IParamMax=[]  DParamMin=[]  DParamMax=[]  NParamMin=[]  NParamMax=[]  KbParamMin=[]  KbParamMax=[]  KtParamMin=[]  KtParamMax=[]  KbOutMin=[]  KbOutMax=[]  KtOutMin=[]  KtOutMax=[]  IntegratorOutMin=[]  IntegratorOutMax=[]  FilterOutMin=[]  FilterOutMax=[]  SumI1OutMin=[]  SumI1OutMax=[]  SumI2OutMin=[]  SumI2OutMax=[]  SumI3OutMin=[]  SumI3OutMax=[]  SumI4OutMin=[]  SumI4OutMax=[]  SumDOutMin=[]  SumDOutMax=[]  DifferentiatorOutMin=[]  DifferentiatorOutMax=[]  FilterDiffOutCoefMin=[]  FilterDiffOutCoefMax=[]  ReciprocalOutMin=[]  ReciprocalOutMax=[]  SumDenOutMin=[]  SumDenOutMax=[]  SumNumOutMin=[]  SumNumOutMax=[]  DivideOutMin=[]  DivideOutMax=[]  UdiffTsProdOutMin=[]  UdiffTsProdOutMax=[]  NTsProdOutMin=[]  NTsProdOutMax=[]  UintegralTsProdOutMin=[]  UintegralTsProdOutMax=[]  UngainTsProdOutMin=[]  UngainTsProdOutMax=[]  IntegratorContinuousStateAttributes=''  IntegratorStateMustResolveToSignalObject=off  IntegratorRTWStateStorageClass=Auto  FilterContinuousStateAttributes=''  FilterStateMustResolveToSignalObject=off  FilterRTWStateStorageClass=Auto  ParallelPVariant=InternalParameters  IdealPVariant=Disabled  IVariant=InternalParameters  DVariant=InternalParameters  IntegratorVariant=Discrete  SatVariant=Disabled  AWVariant=Passthrough  PCopyVariant=Disabled  TRVariant=Disabled  FdbkBlocksVariant=Forward  IdealPFdbkVariant=Disabled  SatFdbkVariant=Disabled  DerivativeFilterVariant=ForwardEulerFilter  NVariant=InternalParameters  NCopyVariant=Disabled  FilterICVariant=InternalICsFilter  IntegratorICVariant=InternalICs  ExternalResetVariant=Disabled  TRSumVariant=Passthrough  SumFdbkVariant=Disabled  SumVariant=Sum_PID  TsampFilterVariant=InternalTs  TsampNgainVariant=Passthrough  TsampIntegralVariant=Disabled_SignalSpec  ExternalSaturationOutDataTypeStr=Inherit: Same as second input
  PLL (3ph)1 : spsPLL3phLib/PLL (3ph)  Fmin=45  Par_Init=[0, 50]  ParK=[180, 3200, 1]  TcD=1e-4  MaxRateChangeFreq=12  FilterCutOffFreq=25  Ts=0  AGC=on
  SVPWM Generator (2-Level)1 : spsSVPWMGenerator2LevelLib/SVPWM Generator (2-Level)  InputType=alpha-beta components  SwitchingPattern=Pattern #1  Fc=10000  ParUref=[0.8 -30 50]  Ts=0
  Scope : Scope  NumInputPorts=2
  Scope1 : Scope  NumInputPorts=2
  Sum1 : Sum  Commented=on  Inputs=|+-
  Sum5 : Sum  Inputs=|+-
  Sum6 : Sum  Inputs=|+-
  Sum7 : Sum  Inputs=++-
  Sum8 : Sum  Inputs=-+|
  Sum9 : Sum  Inputs=+++
  Terminator2 : Terminator
  Terminator3 : Terminator
  Terminator4 : Terminator
  abc to dq1 : spsabctodq0Lib/abc to dq0  Alignment=90 degrees behind phase A axis
  abc to dq2 : spsabctodq0Lib/abc to dq0  Alignment=90 degrees behind phase A axis
  dq0 to Alpha-Beta-Zero1 : spsdq0toAlphaBetaZeroLib/dq0 to Alpha-Beta-Zero  Alignment=90 degrees behind phase A axis
  iq*=0 : Constant  Value=0
  Pulse : Outport
  wires:
  Sum5/1 -> PID 3/1
  Gain6/1 -> Sum7/3
  Demux2/1 -> Sum7/1  "Vd"
  PID 3/1 -> Scope1/1, Sum6/1  "id*"
  dq0 to Alpha-Beta-Zero1/1 -> Gain9/1
  PLL (3ph)1/2 -> dq0 to Alpha-Beta-Zero1/2, abc to dq2/2, abc to dq1/2
  Sum6/1 -> PID 4/1
  PID 4/1 -> Sum7/2
  Demux4/3 -> Terminator4/1
  PID 5/1 -> Sum9/2
  Iabc/1 -> abc to dq2/1
  Constant4/1 -> Mux1/3
  Demux3/3 -> Terminator3/1
  abc to dq1/1 -> Demux2/1
  Demux2/3 -> Terminator2/1
  Udc/1 -> Sum5/1
  abc to dq2/1 -> Demux3/1
  iq*=0/1 -> Scope/2, Sum8/2
  SVPWM Generator (2-Level)1/1 -> Pulse/1
  Gain9/1 -> Demux4/1
  Demux3/2 -> Scope/1, Sum8/1, Gain6/1  "iq"
  Demux3/1 -> Gain7/1, Scope1/2, Sum6/2  "id"
  Sum7/1 -> Mux1/1  "Ud*"
  Sum8/1 -> PID 5/1
  Sum9/1 -> Mux1/2  "Uq*"
  Mux1/1 -> dq0 to Alpha-Beta-Zero1/1
  Demux4/1 -> SVPWM Generator (2-Level)1/1
  Demux4/2 -> SVPWM Generator (2-Level)1/2
  Udc_ref/1 -> Sum5/2
  Gain7/1 -> Sum9/3
  Demux2/2 -> Sum9/1  "Vq"
  Vabc/1 -> PLL (3ph)1/1, abc to dq1/1  "d"
  Constant/1 -> Sum1/2
